simulink model "displayTest"  (R2022b)
settings: Solver=FixedStepDiscrete  StartTime=0.0  StopTime=10.0  FixedStep=0.01  RelTol=1e-3  EnableMultiTasking=on
PreLoadFcn:
  | try, model_open; catch, disp('Error occurred while executing model pre-load callback: model_open.m'); disp('Please assure that the MATLAB working directory is set to the model directory before opening.'); end
InitFcn:
  | try, model_open; catch, end
model workspace (MAT data in the model file):
  IOScreen_Label_XCoord = 1
  IOScreen_Row1_YCoord = 1
  IOScreen_Row2_YCoord = 12
  IOScreen_Value_XCoord = 110
  MainScreen_Row1_YCoord = 7
  MainScreen_Row2_YCoord = 23
  MainScreen_Symbols_XCoord = 1
  MainScreen_Units_XCoord = 69
  MainScreen_Value_XCoord = 64
undefined symbols (not defined in the file or in its folder): curr_screen, DISP, gesture, raptor_get_buildNum, raptor_get_safe_string, raptor_hwexp, raptor_xcp_function, Screens, VC500
libraries: Raptor_display_lib x93, Raptor_lib x40, Raptor_Datalogging_lib x10, simulink_extras x3, simulink x2
(part 2 of 3)

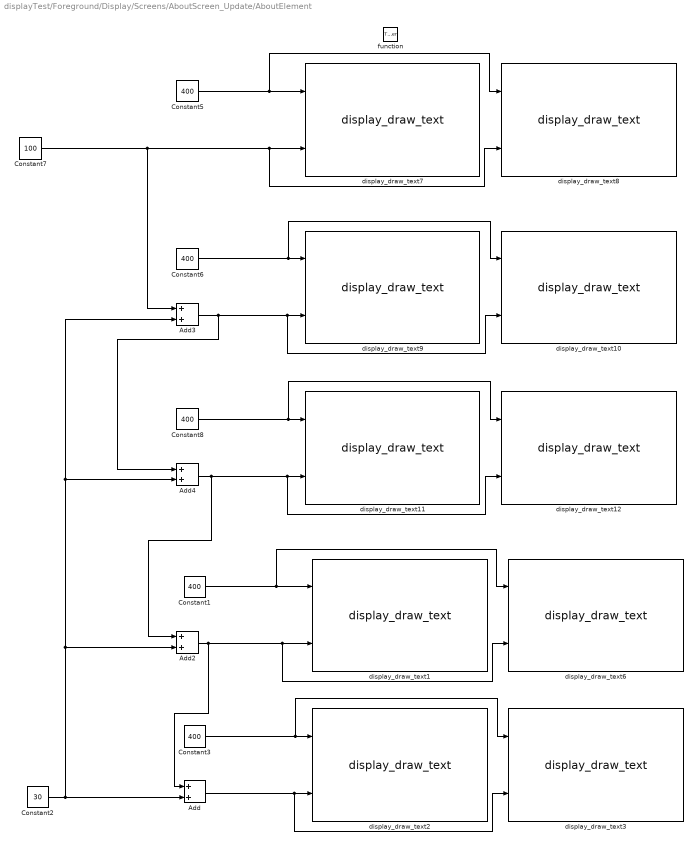
== system displayTest/Foreground/Display/Screens/AboutScreen_Update/AboutElement ==
  function : TriggerPort  TriggerType=function-call  VariantControl=Variant
  Add{,2..4} (4 alike) : Sum
  Constant{1,3,5..6,8} (5 alike) : Constant  Value=400  OutDataTypeStr=int32
  Constant2 : Constant  Value=30  OutDataTypeStr=int32
  Constant7 : Constant  Value=100  OutDataTypeStr=int32
  display_draw_text1 : Raptor_display_lib/Drawing Functions/display_draw_text  textPort=off  textVal='Raptor Version : '  colorPort=off  col=FFFF  opacity=100  font=Future  fontFile=''  heightPort=off  height=20  hAlign=Right  vAlign=Top  spacing=0  layer=Background  pnPort=off
      settings: SourceProductName=Raptor Display Library
  display_draw_text10 : Raptor_display_lib/Drawing Functions/display_draw_text  textPort=off  textVal=get_param(bdroot, 'ModelVersion')  colorPort=off  col=FFFF  opacity=100  font=Future  fontFile=''  heightPort=off  height=20  hAlign=Left  vAlign=Top  spacing=0  layer=Background  pnPort=off
      settings: SourceProductName=Raptor Display Library
  display_draw_text11 : Raptor_display_lib/Drawing Functions/display_draw_text  textPort=off  textVal='Build Number : '  colorPort=off  col=FFFF  opacity=100  font=Future  fontFile=''  heightPort=off  height=20  hAlign=Right  vAlign=Top  spacing=0  layer=Background  pnPort=off
      settings: SourceProductName=Raptor Display Library
  display_draw_text12 : Raptor_display_lib/Drawing Functions/display_draw_text  textPort=off  textVal=num2str(raptor_get_buildNum(bdroot(gcb)))  colorPort=off  col=FFFF  opacity=100  font=Future  fontFile=''  heightPort=off  height=20  hAlign=Left  vAlign=Top  spacing=0  layer=Background  pnPort=off
      settings: SourceProductName=Raptor Display Library
  display_draw_text2 : Raptor_display_lib/Drawing Functions/display_draw_text  textPort=off  textVal='MATLAB Version : '  colorPort=off  col=FFFF  opacity=100  font=Future  fontFile=''  heightPort=off  height=20  hAlign=Right  vAlign=Top  spacing=0  layer=Background  pnPort=off
      settings: SourceProductName=Raptor Display Library
  display_draw_text3 : Raptor_display_lib/Drawing Functions/display_draw_text  textPort=off  textVal=version  colorPort=off  col=FFFF  opacity=100  font=Future  fontFile=''  heightPort=off  height=20  hAlign=Left  vAlign=Top  spacing=0  layer=Background  pnPort=off
      settings: SourceProductName=Raptor Display Library
  display_draw_text6 : Raptor_display_lib/Drawing Functions/display_draw_text  textPort=off  textVal=raptor_hwexp('COMMAND:RAPTOR_VERSION')  colorPort=off  col=FFFF  opacity=100  font=Future  fontFile=''  heightPort=off  height=20  hAlign=Left  vAlign=Top  spacing=0  layer=Background  pnPort=off
      settings: SourceProductName=Raptor Display Library
  display_draw_text7 : Raptor_display_lib/Drawing Functions/display_draw_text  textPort=off  textVal='Application Name : '  colorPort=off  col=FFFF  opacity=100  font=Future  fontFile=''  heightPort=off  height=20  hAlign=Right  vAlign=Top  spacing=0  layer=Background  pnPort=off
      settings: SourceProductName=Raptor Display Library
  display_draw_text8 : Raptor_display_lib/Drawing Functions/display_draw_text  textPort=off  textVal=bdroot  colorPort=off  col=FFFF  opacity=100  font=Future  fontFile=''  heightPort=off  height=20  hAlign=Left  vAlign=Top  spacing=0  layer=Background  pnPort=off
      settings: SourceProductName=Raptor Display Library
  display_draw_text9 : Raptor_display_lib/Drawing Functions/display_draw_text  textPort=off  textVal='Model Version : '  colorPort=off  col=FFFF  opacity=100  font=Future  fontFile=''  heightPort=off  height=20  hAlign=Right  vAlign=Top  spacing=0  layer=Background  pnPort=off
      settings: SourceProductName=Raptor Display Library
  wires:
  Constant1/1 -> display_draw_text6/1, display_draw_text1/1
  Add/1 -> display_draw_text2/2, display_draw_text3/2
  Constant3/1 -> display_draw_text2/1, display_draw_text3/1
  Constant5/1 -> display_draw_text7/1, display_draw_text8/1
  Add2/1 -> Add/1, display_draw_text6/2, display_draw_text1/2
  Constant2/1 -> Add3/2, Add4/2, Add2/2, Add/2
  Add4/1 -> Add2/1, display_draw_text11/2, display_draw_text12/2
  Constant8/1 -> display_draw_text11/1, display_draw_text12/1
  Add3/1 -> Add4/1, display_draw_text9/2, display_draw_text10/2
  Constant6/1 -> display_draw_text9/1, display_draw_text10/1
  Constant7/1 -> display_draw_text7/2, display_draw_text8/2, Add3/1

== system displayTest/Foreground/Display/Screens/DataLogScreen_Create/DataLogScreenSwipe ==
  note: This function is called when a swipe action occurs.  The gesture input will
      |  provide the gesture detected:
      |   0 = UP
      |   1 = DOWN
      |   2 = LEFT
      |   3 = RIGHT
  DataLogScreenSwipe : TriggerPort  TriggerType=function-call  IsSimulinkFunction=on  FunctionName=DataLogScreenSwipe  FunctionVisibility=scoped  VariantControl=Variant  PortDimensions=1
  Constant : Constant  Value=3  OutDataTypeStr=uint8
  Function Caller : FunctionCaller  FunctionPrototype=Screens.Navigation(gesture,curr_screen)  InputArgumentSpecifications=<Enter example>  OutputArgumentSpecifications=<Enter example>
  gesture : ArgIn  OutDataTypeStr=uint8  ArgumentName=gesture
  wires:
  gesture/1 -> Function Caller/1
  Constant/1 -> Function Caller/2

== system displayTest/Foreground/Display/Screens/DataLogScreen_CurrentScreen/EjectButtonPressed ==
  Trigger : TriggerPort  TriggerType=falling  VariantControl=Variant  PortDimensions=1
  raptor_fileIO_USBEject : Raptor_Datalogging_lib/raptor_fileIO_USBEject  variable=0
      settings: SourceProductName=Raptor Data Logging

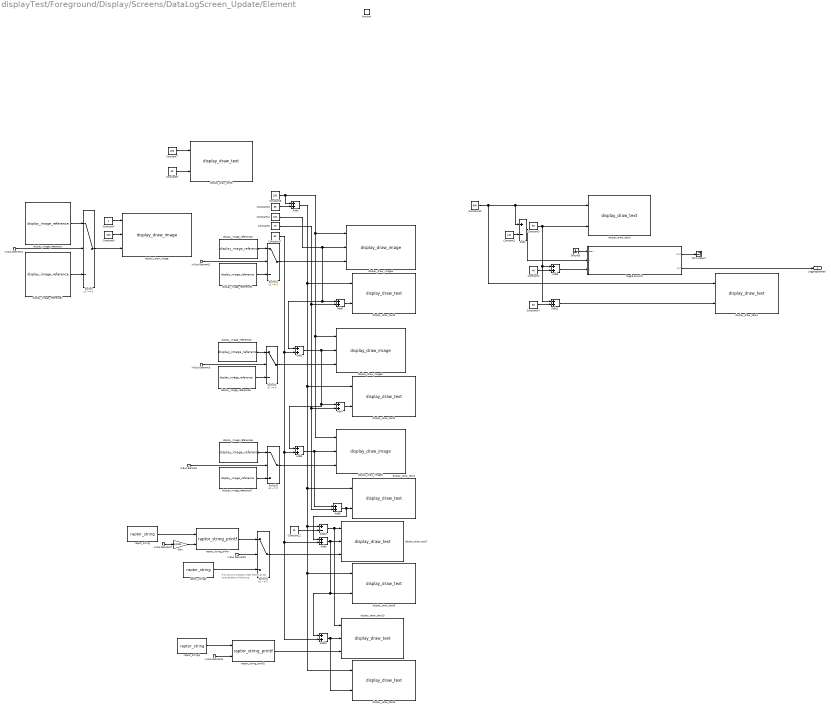
== system displayTest/Foreground/Display/Screens/DataLogScreen_Update/Element ==
  note: If no drive is present, then there can
      | be no evaluation of the size
  In Bus Element2 : Inport  PortName=DataLogState  Element=LoggingPossible
  In Bus Element3 : Inport  PortName=DataLogState  Element=LoggingActive
  In Bus Element : Inport  PortName=DataLogState  Element=EjectReady
  In Bus Element1 : Inport  PortName=DataLogState  Element=USBInserted
  In Bus Element5 : Inport  PortName=DataLogState  Element=USBInserted
  In Bus Element4 : Inport  PortName=DataLogState  Element=LogCounter
  In Bus Element7 : Inport  Port=2  PortName=Sensors  Element=USBFreeSpace
  function : TriggerPort  TriggerType=function-call  VariantControl=Variant
  Add{1,3..9,11,13} (10 alike) : Sum
  Add10 : Sum  Inputs=+-
  Add2 : Sum  Inputs=+-
  Constant1 : Constant  Value=140  OutDataTypeStr=int32
  Constant10 : Constant  Value=600  OutDataTypeStr=int32
  Constant11 : Constant  Value=100  OutDataTypeStr=int32
  Constant12 : Constant  Value=15  OutDataTypeStr=int32
  Constant13 : Constant  Value=65  OutDataTypeStr=int32
  Constant14 : Constant  Value=50  OutDataTypeStr=int32
  Constant17 : Constant  Value=60  OutDataTypeStr=int32
  Constant2 : Constant  Value=40  OutDataTypeStr=int32
  Constant3 : Constant  Value=50  OutDataTypeStr=int32
  Constant4 : Constant  OutDataTypeStr=int32
  Constant5 : Constant  Value=19  OutDataTypeStr=int32
  Constant6 : Constant  Value=100  OutDataTypeStr=int32
  Constant7 : Constant  Value=200  OutDataTypeStr=int32
  Constant8 : Constant  Value=150  OutDataTypeStr=int32
  Constant9 : Constant  Value=50  OutDataTypeStr=int32
  Gain : Gain  Gain=1/1024  OutDataTypeStr=uint32
  Ground3 : Ground
  Switch{,1..4} (5 alike) : Switch  Criteria=u2 ~= 0  SaturateOnIntegerOverflow=off  InputSameDT=off
  Terminator2 : Terminator
  Toggle Switch1 : Subsystem  mask(Display Toggle){InitialCondition=0}
      mask prompts: InitialCondition "Initial Condition"
      mask help: Draws a toggle switch onto the screen that will hold either an off or an on state
      mask Help: eval('raptor_display_help(''Toggle Switch'');')
      mask Display:
      | header = 'Toggle Switch';
      | drawNEBackGndDisplay;
      | port_label('input', 1, 'prev');
      | port_label('input', 2, 'x[int32]');
      | port_label('input', 3, 'y[int32]');
      | port_label('output', 1, 'next');
      | port_label('output', 2, 'out[boolean]');
      | 
      | image(imread('toggle_frame.png'), [0.3 0.2 0.3 0.34]);
  display_draw_image{,1..3} (4 alike) : Raptor_display_lib/Drawing Functions/display_draw_image  imagePort=on  imageFile=USB_Icon_Sprite_Green_25perc.png  opacityPort=off  opacity=100  drawMode=Draw Entire Image  alpha=Draw as Transparent  layer=Background  drawModeXY=Top Left  pnPort=off
      settings: SourceProductName=Raptor Display Library
  display_draw_text1 : Raptor_display_lib/Drawing Functions/display_draw_text  textPort=off  textVal='Ready to Eject'  colorPort=off  col=FFFF  opacity=100  font=Future  fontFile=''  heightPort=off  height=20  hAlign=Left  vAlign=Top  spacing=0  layer=Background  pnPort=off
      settings: SourceProductName=Raptor Display Library
  display_draw_text10 : Raptor_display_lib/Drawing Functions/display_draw_text  textPort=on  textVal='Eject Ready'  colorPort=off  col=FFFF  opacity=100  font=Future  fontFile=''  heightPort=off  height=20  hAlign=Right  vAlign=Top  spacing=0  layer=Background  pnPort=off
      settings: SourceProductName=Raptor Display Library
  display_draw_text2 : Raptor_display_lib/Drawing Functions/display_draw_text  textPort=off  textVal='Control'  colorPort=off  col=FFFF  opacity=100  font=Future  fontFile=''  heightPort=off  height=30  hAlign=Center  vAlign=Top  spacing=0  layer=Background  pnPort=off
      settings: SourceProductName=Raptor Display Library
  display_draw_text3 : Raptor_display_lib/Drawing Functions/display_draw_text  textPort=off  textVal='Logging Active'  colorPort=off  col=FFFF  opacity=100  font=Future  fontFile=''  heightPort=off  height=20  hAlign=Left  vAlign=Top  spacing=0  layer=Background  pnPort=off
      settings: SourceProductName=Raptor Display Library
  display_draw_text4 : Raptor_display_lib/Drawing Functions/display_draw_text  textPort=off  textVal='Logging'  colorPort=off  col=FFFF  opacity=100  font=Future  fontFile=''  heightPort=off  height=20  hAlign=Left  vAlign=Top  spacing=0  layer=Background  pnPort=off
      settings: SourceProductName=Raptor Display Library
  display_draw_text5 : Raptor_display_lib/Drawing Functions/display_draw_text  textPort=off  textVal='Ready to Log'  colorPort=off  col=FFFF  opacity=100  font=Future  fontFile=''  heightPort=off  height=20  hAlign=Left  vAlign=Top  spacing=0  layer=Background  pnPort=off
      settings: SourceProductName=Raptor Display Library
  display_draw_text6 : Raptor_display_lib/Drawing Functions/display_draw_text  textPort=off  textVal='USB Free Space'  colorPort=off  col=FFFF  opacity=100  font=Future  fontFile=''  heightPort=off  height=20  hAlign=Left  vAlign=Top  spacing=0  layer=Background  pnPort=off
      settings: SourceProductName=Raptor Display Library
  display_draw_text7 : Raptor_display_lib/Drawing Functions/display_draw_text  textPort=on  textVal='Eject Ready'  colorPort=off  col=FFFF  opacity=100  font=Future  fontFile=''  heightPort=off  height=20  hAlign=Right  vAlign=Top  spacing=0  layer=Background  pnPort=off
      settings: SourceProductName=Raptor Display Library
  display_draw_text8 : Raptor_display_lib/Drawing Functions/display_draw_text  textPort=off  textVal='Status'  colorPort=off  col=FFFF  opacity=100  font=Future  fontFile=''  heightPort=off  height=30  hAlign=Center  vAlign=Top  spacing=0  layer=Background  pnPort=off
      settings: SourceProductName=Raptor Display Library
  display_draw_text9 : Raptor_display_lib/Drawing Functions/display_draw_text  textPort=off  textVal='# Lines Logged'  colorPort=off  col=FFFF  opacity=100  font=Future  fontFile=''  heightPort=off  height=20  hAlign=Left  vAlign=Top  spacing=0  layer=Background  pnPort=off
      settings: SourceProductName=Raptor Display Library
  display_image_reference : Raptor_display_lib/Drawing Functions/display_image_reference  imageFile=USB_Icon_Sprite_Green_25perc.png
      settings: SourceProductName=Raptor Display Library
  display_image_reference1 : Raptor_display_lib/Drawing Functions/display_image_reference  imageFile=USB_Icon_Sprite_Red_25perc.png
      settings: SourceProductName=Raptor Display Library
  display_image_reference2 : Raptor_display_lib/Drawing Functions/display_image_reference  imageFile=Oval Driver@2x.png
      settings: SourceProductName=Raptor Display Library
  display_image_reference3 : Raptor_display_lib/Drawing Functions/display_image_reference  imageFile=Oval Active@2x.png
      settings: SourceProductName=Raptor Display Library
  display_image_reference4 : Raptor_display_lib/Drawing Functions/display_image_reference  imageFile=Oval Driver@2x.png
      settings: SourceProductName=Raptor Display Library
  display_image_reference5 : Raptor_display_lib/Drawing Functions/display_image_reference  imageFile=Oval Active@2x.png
      settings: SourceProductName=Raptor Display Library
  display_image_reference6 : Raptor_display_lib/Drawing Functions/display_image_reference  imageFile=Oval Driver@2x.png
      settings: SourceProductName=Raptor Display Library
  display_image_reference7 : Raptor_display_lib/Drawing Functions/display_image_reference  imageFile=Oval Active@2x.png
      settings: SourceProductName=Raptor Display Library
  raptor_string : Raptor_lib/Strings/raptor_string  stringName=''  string=''  dynamicSize=Fixed Size  strSize=20  storage=Volatile (RAM)  calVisible=off  calAccess=4  strFunction=raptor_xcp_function(gcb)
      settings: SourceProductName=Raptor
  raptor_string1 : Raptor_lib/Strings/raptor_string  stringName=''  string=''  dynamicSize=Fixed Size  strSize=20  storage=Volatile (RAM)  calVisible=off  calAccess=4  strFunction=raptor_xcp_function(gcb)
      settings: SourceProductName=Raptor
  raptor_string2 : Raptor_lib/Strings/raptor_string  stringName=''  string='N/A'  dynamicSize=Size from initial value  strSize=20  storage=Volatile (RAM)  calVisible=off  calAccess=4  strFunction=raptor_xcp_function(gcb)
      settings: SourceProductName=Raptor
  raptor_string_printf : Raptor_lib/Strings/raptor_string_printf  formatString='%u KB'
      settings: SourceProductName=Raptor
  raptor_string_printf1 : Raptor_lib/Strings/raptor_string_printf  formatString='%u'
      settings: SourceProductName=Raptor
  LoggingEnabled : Outport  VectorParamsAs1DForOutWhenUnconnected=off
  wires:
  Constant2/1 -> Add3/2
  Add2/1 -> Toggle Switch1/2(x)
  Toggle Switch1/1(next) -> Terminator2/1
  Toggle Switch1/2(out) -> LoggingEnabled/1
  Ground3/1 -> Toggle Switch1/1(prev)
  Constant10/1 -> display_draw_text4/1, Add2/1, display_draw_text2/1
  Constant1/1 -> Add2/2
  Add3/1 -> Toggle Switch1/3(y)
  Constant6/1 -> display_draw_image/2
  Constant4/1 -> display_draw_image/1
  display_image_reference/1 -> Switch/1
  display_image_reference1/1 -> Switch/3
  In Bus Element1/1 -> Switch/2
  Switch/1 -> display_draw_image/3
  Switch1/1 -> display_draw_image1/3
  Constant8/1 -> Add4/1, display_draw_image3/1, display_draw_image2/1, display_draw_image1/1
  Constant11/1 -> Add1/1, Add6/1, display_draw_image1/2
  Add1/1 -> Add7/1, Add5/1, display_draw_image2/2
  Switch2/1 -> display_draw_image2/3
  Switch3/1 -> display_draw_image3/3
  display_image_reference7/1 -> Switch3/3
  display_image_reference6/1 -> Switch3/1
  In Bus Element/1 -> Switch3/2
  Constant13/1 -> Add4/2
  Constant17/1 -> Add13/2, Add9/2, Add5/2, Add1/2
  Add5/1 -> Add8/1, display_draw_image3/2
  Constant5/1 -> Add8/2, Add7/2, Add6/2
  Add6/1 -> display_draw_text5/2
  Add7/1 -> display_draw_text3/2
  Add8/1 -> Add9/1, display_draw_text1/2
  raptor_string/1 -> raptor_string_printf/1
  In Bus Element7/1 -> Gain/1
  Constant7/1 -> display_draw_text8/1
  Constant9/1 -> display_draw_text8/2
  Constant12/1 -> Add10/2
  Constant3/1 -> Add11/1, Add3/1, display_draw_text2/2
  Add10/1 -> display_draw_text10/1, display_draw_text7/1
  Add13/1 -> display_draw_text10/2, display_draw_text9/2
  raptor_string_printf1/1 -> display_draw_text10/3
  In Bus Element4/1 -> raptor_string_printf1/2
  raptor_string1/1 -> raptor_string_printf1/1
  Add9/1 -> Add13/1, display_draw_text6/2, display_draw_text7/2
  Add4/1 -> display_draw_text5/1, Add10/1, display_draw_text9/1, display_draw_text6/1, display_draw_text1/1, display_draw_text3/1
  raptor_string_printf/1 -> Switch4/1
  Switch4/1 -> display_draw_text7/3
  raptor_string2/1 -> Switch4/3
  In Bus Element5/1 -> Switch4/2
  Gain/1 -> raptor_string_printf/2
  In Bus Element3/1 -> Switch2/2
  display_image_reference4/1 -> Switch2/1
  display_image_reference5/1 -> Switch2/3
  display_image_reference3/1 -> Switch1/3
  display_image_reference2/1 -> Switch1/1
  In Bus Element2/1 -> Switch1/2
  Add11/1 -> display_draw_text4/2
  Constant14/1 -> Add11/2

== system displayTest/Foreground/Display/Screens/IOScreen_Create/IOScreenSwipe ==
  note: This function is called when a swipe action occurs.  The gesture input will
      |  provide the gesture detected:
      |   0 = UP
      |   1 = DOWN
      |   2 = LEFT
      |   3 = RIGHT
  IOScreenSwipe : TriggerPort  TriggerType=function-call  IsSimulinkFunction=on  FunctionName=IOScreenSwipe  FunctionVisibility=scoped  VariantControl=Variant  PortDimensions=1
  Constant : Constant  Value=2  OutDataTypeStr=uint8
  Function Caller : FunctionCaller  FunctionPrototype=Screens.Navigation(gesture,curr_screen)  InputArgumentSpecifications=<Enter example>  OutputArgumentSpecifications=<Enter example>
  gesture : ArgIn  OutDataTypeStr=uint8  ArgumentName=gesture
  wires:
  Constant/1 -> Function Caller/2
  gesture/1 -> Function Caller/1

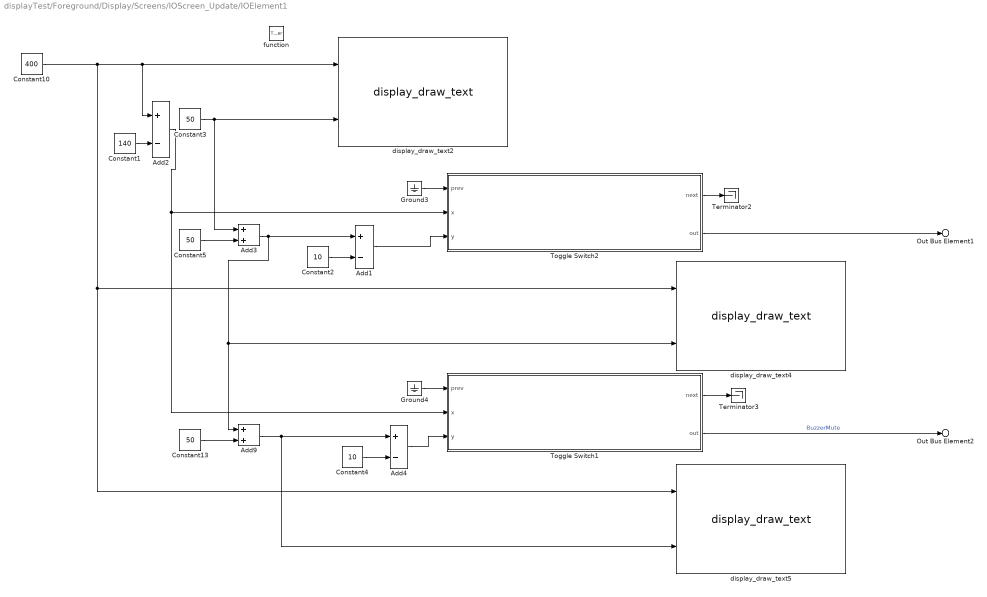
== system displayTest/Foreground/Display/Screens/IOScreen_Update/IOElement1 ==
  function : TriggerPort  TriggerType=function-call  VariantControl=Variant
  Add1 : Sum  Inputs=+-
  Add2 : Sum  Inputs=+-
  Add3 : Sum
  Add4 : Sum  Inputs=+-
  Add9 : Sum
  Constant1 : Constant  Value=140  OutDataTypeStr=int32
  Constant10 : Constant  Value=400  OutDataTypeStr=int32
  Constant13 : Constant  Value=50  OutDataTypeStr=int32
  Constant2 : Constant  Value=10  OutDataTypeStr=int32
  Constant3 : Constant  Value=50  OutDataTypeStr=int32
  Constant4 : Constant  Value=10  OutDataTypeStr=int32
  Constant5 : Constant  Value=50  OutDataTypeStr=int32
  Ground3 : Ground
  Ground4 : Ground
  Terminator2 : Terminator
  Terminator3 : Terminator
  Toggle Switch1 : Subsystem  mask(Display Toggle){InitialCondition=0}
      mask prompts: InitialCondition "Initial Condition"
      mask help: Draws a toggle switch onto the screen that will hold either an off or an on state
      mask Help: eval('raptor_display_help(''Toggle Switch'');')
      mask Display:
      | header = 'Toggle Switch';
      | drawNEBackGndDisplay;
      | port_label('input', 1, 'prev');
      | port_label('input', 2, 'x[int32]');
      | port_label('input', 3, 'y[int32]');
      | port_label('output', 1, 'next');
      | port_label('output', 2, 'out[boolean]');
      | 
      | image(imread('toggle_frame.png'), [0.3 0.2 0.3 0.34]);
  Toggle Switch2 : Subsystem  mask(Display Toggle){InitialCondition=0}
      mask prompts: InitialCondition "Initial Condition"
      mask help: Draws a toggle switch onto the screen that will hold either an off or an on state
      mask Help: eval('raptor_display_help(''Toggle Switch'');')
      mask Display:
      | header = 'Toggle Switch';
      | drawNEBackGndDisplay;
      | port_label('input', 1, 'prev');
      | port_label('input', 2, 'x[int32]');
      | port_label('input', 3, 'y[int32]');
      | port_label('output', 1, 'next');
      | port_label('output', 2, 'out[boolean]');
      | 
      | image(imread('toggle_frame.png'), [0.3 0.2 0.3 0.34]);
  display_draw_text2 : Raptor_display_lib/Drawing Functions/display_draw_text  textPort=off  textVal='Outputs'  colorPort=off  col=FFFF  opacity=100  font=Future  fontFile=''  heightPort=off  height=30  hAlign=Center  vAlign=Top  spacing=0  layer=Background  pnPort=off
      settings: SourceProductName=Raptor Display Library
  display_draw_text4 : Raptor_display_lib/Drawing Functions/display_draw_text  textPort=off  textVal='Buzzer'  colorPort=off  col=FFFF  opacity=100  font=Future  fontFile=''  heightPort=off  height=20  hAlign=Left  vAlign=Top  spacing=0  layer=Background  pnPort=off
      settings: SourceProductName=Raptor Display Library
  display_draw_text5 : Raptor_display_lib/Drawing Functions/display_draw_text  textPort=off  textVal='Buzzer Mute'  colorPort=off  col=FFFF  opacity=100  font=Future  fontFile=''  heightPort=off  height=20  hAlign=Left  vAlign=Top  spacing=0  layer=Background  pnPort=off
      settings: SourceProductName=Raptor Display Library
  Out Bus Element1 : Outport  VectorParamsAs1DForOutWhenUnconnected=off  PortName=Actuators  Element=Buzzer
  Out Bus Element2 : Outport  VectorParamsAs1DForOutWhenUnconnected=off  PortName=Actuators  Element=BuzzerMute
  wires:
  Constant13/1 -> Add9/2
  Ground4/1 -> Toggle Switch1/1(prev)
  Add9/1 -> Add4/1, display_draw_text5/2
  Toggle Switch1/1(next) -> Terminator3/1
  Toggle Switch1/2(out) -> Out Bus Element2/1  "BuzzerMute"
  Toggle Switch2/2(out) -> Out Bus Element1/1
  Toggle Switch2/1(next) -> Terminator2/1
  Ground3/1 -> Toggle Switch2/1(prev)
  Constant10/1 -> Add2/1, display_draw_text2/1, display_draw_text4/1, display_draw_text5/1
  Constant3/1 -> Add3/1, display_draw_text2/2
  Add2/1 -> Toggle Switch2/2(x), Toggle Switch1/2(x)
  Constant1/1 -> Add2/2
  Add3/1 -> Add1/1, display_draw_text4/2, Add9/1
  Constant5/1 -> Add3/2
  Constant2/1 -> Add1/2
  Add1/1 -> Toggle Switch2/3(y)
  Constant4/1 -> Add4/2
  Add4/1 -> Toggle Switch1/3(y)

== system displayTest/Foreground/Display/Screens/MainScreen_Create/MainScreenSwipe ==
  note: This function is called when a swipe action occurs.  The gesture input will
      |  provide the gesture detected:
      |   0 = UP
      |   1 = DOWN
      |   2 = LEFT
      |   3 = RIGHT
  MainScreenSwipe : TriggerPort  TriggerType=function-call  IsSimulinkFunction=on  FunctionName=MainScreenSwipe  FunctionVisibility=scoped  VariantControl=Variant  PortDimensions=1
  Constant : Constant  OutDataTypeStr=uint8
  Function Caller : FunctionCaller  FunctionPrototype=Screens.Navigation(gesture,curr_screen)  InputArgumentSpecifications=<Enter example>  OutputArgumentSpecifications=<Enter example>
  gesture : ArgIn  OutDataTypeStr=uint8  ArgumentName=gesture
  wires:
  gesture/1 -> Function Caller/1
  Constant/1 -> Function Caller/2

== system displayTest/Foreground/Display/Screens/MainScreen_Update/Illumination Invalid ==
  Xbase : Inport
  Ybase : Inport  Port=2
  Prev : Inport  Port=3
  Enable : EnablePort
  Add : Sum
  Add1 : Sum  Inputs=+-
  Constant1 : Constant  Value=51  OutDataTypeStr=int32
  Constant74 : Constant  Value=20  OutDataTypeStr=int32
  Terminator : Terminator
  display_draw_image : Raptor_display_lib/Drawing Functions/display_draw_image  imagePort=off  imageFile=FaultRED.bmp  opacityPort=off  opacity=100  drawMode=Draw Entire Image  alpha=Draw as Transparent  layer=Background  drawModeXY=Top Left  pnPort=on
      settings: SourceProductName=Raptor Display Library
  wires:
  display_draw_image/1 -> Terminator/1
  Prev/1 -> display_draw_image/1
  Add/1 -> display_draw_image/3
  Constant74/1 -> Add/2
  Ybase/1 -> Add/1
  Constant1/1 -> Add1/2
  Xbase/1 -> Add1/1
  Add1/1 -> display_draw_image/2

== system displayTest/Foreground/Display/Screens/MainScreen_Update/RPM Invalid ==
  Xbase : Inport
  Ybase : Inport  Port=2
  Prev : Inport  Port=3
  Enable : EnablePort
  Add : Sum
  Constant74 : Constant  Value=20  OutDataTypeStr=int32
  Terminator : Terminator
  display_draw_image : Raptor_display_lib/Drawing Functions/display_draw_image  imagePort=off  imageFile=FaultRED.bmp  opacityPort=off  opacity=100  drawMode=Draw Entire Image  alpha=Draw as Transparent  layer=Background  drawModeXY=Top Left  pnPort=on
      settings: SourceProductName=Raptor Display Library
  wires:
  Xbase/1 -> display_draw_image/2
  Ybase/1 -> Add/1
  Constant74/1 -> Add/2
  Add/1 -> display_draw_image/3
  Prev/1 -> display_draw_image/1
  display_draw_image/1 -> Terminator/1

== system displayTest/Foreground/Display/Screens/Navigation/Go Left ==
  Current Screen : Inport
  Action Port : ActionPort  ActionPortLabel=elseif(u1 == 2)
  About : Subsystem  TreatAsAtomicUnit=on
  DataLog : Subsystem  TreatAsAtomicUnit=on
  Default : Subsystem  TreatAsAtomicUnit=on
  IO : Subsystem  TreatAsAtomicUnit=on
  Main : Subsystem  TreatAsAtomicUnit=on
  Switch Case1 : SwitchCase  CaseConditions={1,2,3,4}
  wires:
  Switch Case1/2 -> IO/Action
  Switch Case1/5 -> Default/Action
  Switch Case1/4 -> About/Action
  Switch Case1/1 -> Main/Action
  Switch Case1/3 -> DataLog/Action
  Current Screen/1 -> Switch Case1/1

== system displayTest/Foreground/Display/Screens/Navigation/Go Right ==
  Current Screen : Inport
  Action Port : ActionPort  ActionPortLabel=if(u1 == 3)
  About : Subsystem  TreatAsAtomicUnit=on
  DataLog : Subsystem  TreatAsAtomicUnit=on
  Default : Subsystem  TreatAsAtomicUnit=on
  IO : Subsystem  TreatAsAtomicUnit=on
  Main : Subsystem  TreatAsAtomicUnit=on
  Switch Case : SwitchCase  CaseConditions={1,2,3,4}
  wires:
  Current Screen/1 -> Switch Case/1
  Switch Case/1 -> Main/Action
  Switch Case/3 -> DataLog/Action
  Switch Case/4 -> About/Action
  Switch Case/2 -> IO/Action
  Switch Case/5 -> Default/Action

== system displayTest/Foreground/Display/Screens/Navigation/Go Up or Down ==
  note: Do Nothing when a "UP" or "DOWN" is performed
  Current Screen : Inport
  Action Port : ActionPort  ActionPortLabel=else
  Terminator : Terminator
  wires:
  Current Screen/1 -> Terminator/1

== system displayTest/Foreground/Plant/Inputs/J1939 Rx/Process Illumination Message ==
  note: default to 100% illumination
  note: timeout occurred
  note: new message
  AgeCount : Inport
  Data : Inport  Port=2
  Constant : Constant  Value=750
  Constant1 : Constant  Value=0
  Constant2 : Constant  Value=100
  Constant3 : Constant  Value=100
  Logical Operator : Logic  Operator=NOT  AllPortsSameDT=off  OutDataTypeStr=boolean
  Logical Operator1 : Logic  Operator=OR  AllPortsSameDT=off  OutDataTypeStr=boolean
  Relational Operator : RelationalOperator  Operator=>  OutDataTypeStr=boolean  RndMeth=Simplest  InputSameDT=off
  Relational Operator1 : RelationalOperator  Operator===  OutDataTypeStr=boolean  RndMeth=Simplest  InputSameDT=off
  Relational Operator2 : RelationalOperator  Operator=>  OutDataTypeStr=boolean  RndMeth=Simplest  InputSameDT=off
  Switch : Switch  Criteria=u2 ~= 0  SaturateOnIntegerOverflow=off  InputSameDT=off
  Switch1 : Switch  Criteria=u2 ~= 0  SaturateOnIntegerOverflow=off  InputSameDT=off
  Unit Delay : UnitDelay  SampleTime=-1  HasFrameUpgradeWarning=on
  Illumination : Outport  VectorParamsAs1DForOutWhenUnconnected=off
  IlluminationValid : Outport  Port=2  VectorParamsAs1DForOutWhenUnconnected=off
  wires:
  Constant/1 -> Relational Operator/2
  Logical Operator/1 -> IlluminationValid/1
  Switch/1 -> Illumination/1, Unit Delay/1
  AgeCount/1 -> Relational Operator1/1, Relational Operator/1
  Constant1/1 -> Relational Operator1/2
  Relational Operator1/1 -> Switch1/2
  Data/1 -> Switch1/1, Relational Operator2/1
  Switch1/1 -> Switch/3
  Unit Delay/1 -> Switch1/3
  Constant2/1 -> Switch/1
  Relational Operator/1 -> Logical Operator1/1
  Logical Operator1/1 -> Switch/2, Logical Operator/1
  Relational Operator2/1 -> Logical Operator1/2
  Constant3/1 -> Relational Operator2/2

== system displayTest/Foreground/Plant/Inputs/J1939 Rx/Process RPM Message ==
  note: timeout occurred
  note: new message
  AgeCount : Inport
  Data : Inport  Port=2
  Constant : Constant  Value=100
  Constant1 : Constant  Value=0
  Constant2 : Constant  Value=0
  Constant3 : Constant  Value=8031.88
  Logical Operator : Logic  Operator=NOT  AllPortsSameDT=off  OutDataTypeStr=boolean
  Logical Operator1 : Logic  Operator=OR  AllPortsSameDT=off  OutDataTypeStr=boolean
  Relational Operator : RelationalOperator  Operator=>  OutDataTypeStr=boolean  RndMeth=Simplest  InputSameDT=off
  Relational Operator1 : RelationalOperator  Operator===  OutDataTypeStr=boolean  RndMeth=Simplest  InputSameDT=off
  Relational Operator2 : RelationalOperator  Operator=>  OutDataTypeStr=boolean  RndMeth=Simplest  InputSameDT=off
  Switch : Switch  Criteria=u2 ~= 0  SaturateOnIntegerOverflow=off  InputSameDT=off
  Switch1 : Switch  Criteria=u2 ~= 0  SaturateOnIntegerOverflow=off  InputSameDT=off
  Unit Delay : UnitDelay  SampleTime=-1  HasFrameUpgradeWarning=on
  EngineRPM : Outport  VectorParamsAs1DForOutWhenUnconnected=off
  EngineRPMValid : Outport  Port=2  VectorParamsAs1DForOutWhenUnconnected=off
  wires:
  Constant/1 -> Relational Operator/2
  Logical Operator/1 -> EngineRPMValid/1
  Switch/1 -> EngineRPM/1, Unit Delay/1
  AgeCount/1 -> Relational Operator1/1, Relational Operator/1
  Constant1/1 -> Relational Operator1/2
  Relational Operator1/1 -> Switch1/2
  Data/1 -> Switch1/1, Relational Operator2/1
  Switch1/1 -> Switch/3
  Unit Delay/1 -> Switch1/3
  Constant2/1 -> Switch/1
  Relational Operator/1 -> Logical Operator1/1
  Logical Operator1/1 -> Switch/2, Logical Operator/1
  Relational Operator2/1 -> Logical Operator1/2
  Constant3/1 -> Relational Operator2/2

== system displayTest/Foreground/Display/Data Logging/Write to Log/File Write Action/Sync File ==
  In1 : Inport
  Enable : EnablePort
  Terminator : Terminator
  Terminator1 : Terminator
  raptor_data_write : Raptor_lib/Data Storage/raptor_data_write  dataName='LastSync'  dataShape=Scalar  idxSource=Input Port  idxRow=1  idxCol=1
      settings: SourceProductName=Raptor
  raptor_fileIO_sync1 : Raptor_Datalogging_lib/raptor_fileIO_sync  resourceValues=USB|(None)  resource=USB
      settings: SourceProductName=Raptor Data Logging
  raptor_time : Raptor_lib/Triggers/raptor_time  unit=milliseconds
      settings: SourceProductName=Raptor
  wires:
  raptor_time/1 -> raptor_data_write/1
  raptor_fileIO_sync1/1 -> Terminator/1
  In1/1 -> raptor_fileIO_sync1/1
  raptor_fileIO_sync1/2 -> Terminator1/1

== system displayTest/Foreground/Display/Data Logging/Write to Log/File Write Action/Sync every 10 Seconds ==
  Add1 : Sum  Inputs=+-
  Constant : Constant  Value=10000
  Logical Operator : Logic  Operator=OR  AllPortsSameDT=off  OutDataTypeStr=boolean
  Relational Operator : RelationalOperator  Operator=>  OutDataTypeStr=boolean  InputSameDT=off
  Relational Operator1 : RelationalOperator  Operator=<  OutDataTypeStr=boolean  InputSameDT=off
  Unit Delay : UnitDelay  SampleTime=-1  HasFrameUpgradeWarning=on
  raptor_data_def : Raptor_lib/Data Storage/raptor_data_def  dataName='LastSync'  initValue=0  dataType=uint32  storage=Volatile (RAM)  calVisible=on  calType=Measurement  calDispType=Number  calEnum={'False', 'True'}  calGain=1.0  calOffset=0  calMin=-Inf  calMax=Inf  calFormat='4.2'  calUnit=''  calHelp=['Block:' gcb]  calAccess=4  calFunction=raptor_xcp_function(gcb)  calDispHeaders=off  calColHeaders={'Col1' 'Col2' 'Col3'}  calRowHeaders={'Row1' 'Row2' 'Row3'}
      settings: SourceProductName=Raptor
  raptor_data_read1 : Raptor_lib/Data Storage/raptor_data_read  dataName='LastSync'  dataShape=Scalar  idxSource=Input  idxRow=1  idxCol=1
      settings: SourceProductName=Raptor
  raptor_time : Raptor_lib/Triggers/raptor_time  unit=milliseconds
      settings: SourceProductName=Raptor
  TimeToSync : Outport  VectorParamsAs1DForOutWhenUnconnected=off
  wires:
  Logical Operator/1 -> TimeToSync/1
  Relational Operator1/1 -> Logical Operator/2  "Rollover"
  Relational Operator/1 -> Logical Operator/1
  Constant/1 -> Relational Operator/2
  Add1/1 -> Relational Operator/1
  raptor_data_read1/1 -> Add1/2
  Unit Delay/1 -> Relational Operator1/2
  raptor_time/1 -> Relational Operator1/1, Add1/1, Unit Delay/1

== system displayTest/Foreground/Display/Data Logging/Write to Log/Open Existing File/File Seek ==
  Open File Handle : Inport
  Open Success : Inport  Port=2
  File Open Failure : Subsystem
  File Open Success : Subsystem
  Logical Operator : Logic  Operator=NOT  AllPortsSameDT=off  OutDataTypeStr=boolean
  Seek File Handle Success : Outport  VectorParamsAs1DForOutWhenUnconnected=off
  Seek Success : Outport  Port=2  VectorParamsAs1DForOutWhenUnconnected=off
  Seek File Handle Failure : Outport  Port=3  VectorParamsAs1DForOutWhenUnconnected=off
  Seek Failure : Outport  Port=4  VectorParamsAs1DForOutWhenUnconnected=off
  wires:
  Open File Handle/1 -> File Open Success/1(file_in), File Open Failure/1(file_in)
  Logical Operator/1 -> File Open Failure/Enable
  Open Success/1 -> Logical Operator/1, File Open Success/Enable
  File Open Success/1(file_out) -> Seek File Handle Success/1
  File Open Success/2(Out2) -> Seek Success/1
  File Open Failure/1(file_out) -> Seek File Handle Failure/1
  File Open Failure/2(Success) -> Seek Failure/1

== system displayTest/Foreground/Display/Data Logging/Write to Log/Open Existing File/Merge ==
  File Handle Success : Inport
  File Open Success : Inport  Port=2
  File Handle Failure : Inport  Port=3
  File Open Failure : Inport  Port=4
  Merge : Merge
  Merge1 : Merge
  Handle : Outport  VectorParamsAs1DForOutWhenUnconnected=off
  Success : Outport  Port=2  VectorParamsAs1DForOutWhenUnconnected=off
  wires:
  Merge1/1 -> Handle/1
  Merge/1 -> Success/1
  File Open Failure/1 -> Merge/2
  File Handle Failure/1 -> Merge1/2
  File Handle Success/1 -> Merge1/1
  File Open Success/1 -> Merge/1

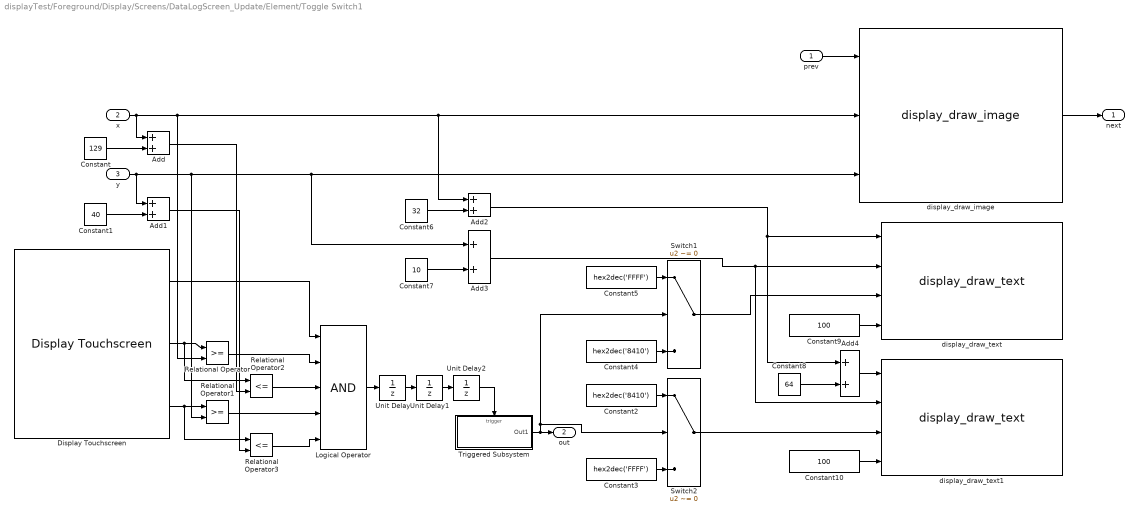
== system displayTest/Foreground/Display/Screens/DataLogScreen_Update/Element/Toggle Switch1 ==
  prev : Inport
  x : Inport  Port=2
  y : Inport  Port=3
  Add{,1..4} (5 alike) : Sum
  Constant : Constant  Value=129
  Constant1 : Constant  Value=40
  Constant10 : Constant  Value=100  OutDataTypeStr=uint32
  Constant2 : Constant  Value=hex2dec('8410')  OutDataTypeStr=uint16
  Constant3 : Constant  Value=hex2dec('FFFF')  OutDataTypeStr=uint16
  Constant4 : Constant  Value=hex2dec('8410')  OutDataTypeStr=uint16
  Constant5 : Constant  Value=hex2dec('FFFF')  OutDataTypeStr=uint16
  Constant6 : Constant  Value=32  OutDataTypeStr=int32
  Constant7 : Constant  Value=10  OutDataTypeStr=int32
  Constant8 : Constant  Value=64  OutDataTypeStr=int32
  Constant9 : Constant  Value=100  OutDataTypeStr=uint32
  Display Touchscreen : Raptor_display_lib/Touchscreen/Display Touchscreen
      settings: SourceProductName=Raptor Display Library
  Logical Operator : Logic  Inputs=5  IconShape=distinctive  AllPortsSameDT=off  OutDataTypeStr=boolean
  Relational Operator : RelationalOperator  OutDataTypeStr=boolean  InputSameDT=off
  Relational Operator1 : RelationalOperator  OutDataTypeStr=boolean  InputSameDT=off
  Relational Operator2 : RelationalOperator  Operator=<=  OutDataTypeStr=boolean  InputSameDT=off
  Relational Operator3 : RelationalOperator  Operator=<=  OutDataTypeStr=boolean  InputSameDT=off
  Switch1 : Switch  Criteria=u2 ~= 0  SaturateOnIntegerOverflow=off  InputSameDT=off
  Switch2 : Switch  Criteria=u2 ~= 0  SaturateOnIntegerOverflow=off  InputSameDT=off
  Triggered Subsystem : Subsystem  TreatAsAtomicUnit=on
  Unit Delay : UnitDelay  SampleTime=-1  HasFrameUpgradeWarning=on
  Unit Delay1 : UnitDelay  InitialCondition=1  SampleTime=-1  HasFrameUpgradeWarning=on
  Unit Delay2 : UnitDelay  SampleTime=-1  HasFrameUpgradeWarning=on
  display_draw_image : Raptor_display_lib/Drawing Functions/display_draw_image  imagePort=off  imageFile=toggle_frame.png  opacityPort=off  opacity=100  drawMode=Draw Entire Image  alpha=Draw as Transparent  layer=Background  drawModeXY=Top Left  pnPort=on
      settings: SourceProductName=Raptor Display Library
  display_draw_text : Raptor_display_lib/Drawing Functions/display_draw_text  textPort=off  textVal='On'  colorPort=on  col=8410  opacity=100  font=Future  fontFile=''  heightPort=off  height=20  hAlign=Center  vAlign=Top  spacing=0  layer=Background  pnPort=off
      settings: SourceProductName=Raptor Display Library
  display_draw_text1 : Raptor_display_lib/Drawing Functions/display_draw_text  textPort=off  textVal='Off'  colorPort=on  col=FFFF  opacity=100  font=Future  fontFile=''  heightPort=off  height=20  hAlign=Center  vAlign=Top  spacing=0  layer=Background  pnPort=off
      settings: SourceProductName=Raptor Display Library
  next : Outport  VectorParamsAs1DForOutWhenUnconnected=off
  out : Outport  Port=2  VectorParamsAs1DForOutWhenUnconnected=off
  wires:
  x/1 -> Add/1, Relational Operator/2, Add2/1, display_draw_image/2
  Display Touchscreen/2 -> Relational Operator/1, Relational Operator2/1
  Display Touchscreen/3 -> Relational Operator1/1, Relational Operator3/1
  y/1 -> Add1/1, Relational Operator1/2, Add3/1, display_draw_image/3
  Constant/1 -> Add/2
  Constant1/1 -> Add1/2
  Add/1 -> Relational Operator2/2
  Add1/1 -> Relational Operator3/2
  Relational Operator3/1 -> Logical Operator/5
  Relational Operator1/1 -> Logical Operator/4
  Relational Operator2/1 -> Logical Operator/3
  Relational Operator/1 -> Logical Operator/2
  Display Touchscreen/1 -> Logical Operator/1
  Unit Delay1/1 -> Unit Delay2/1
  Unit Delay/1 -> Unit Delay1/1
  Logical Operator/1 -> Unit Delay/1
  Unit Delay2/1 -> Triggered Subsystem/Trigger
  prev/1 -> display_draw_image/1
  display_draw_image/1 -> next/1
  Triggered Subsystem/1(Out1) -> Switch1/2, Switch2/2, out/1
  Switch1/1 -> display_draw_text/3
  Switch2/1 -> display_draw_text1/3
  Constant2/1 -> Switch2/1
  Constant4/1 -> Switch1/3
  Constant3/1 -> Switch2/3
  Constant5/1 -> Switch1/1
  Constant6/1 -> Add2/2
  Add2/1 -> Add4/1, display_draw_text/1
  Constant7/1 -> Add3/2
  Add3/1 -> display_draw_text/2, display_draw_text1/2
  Constant8/1 -> Add4/2
  Add4/1 -> display_draw_text1/1
  Constant9/1 -> display_draw_text/4
  Constant10/1 -> display_draw_text1/4

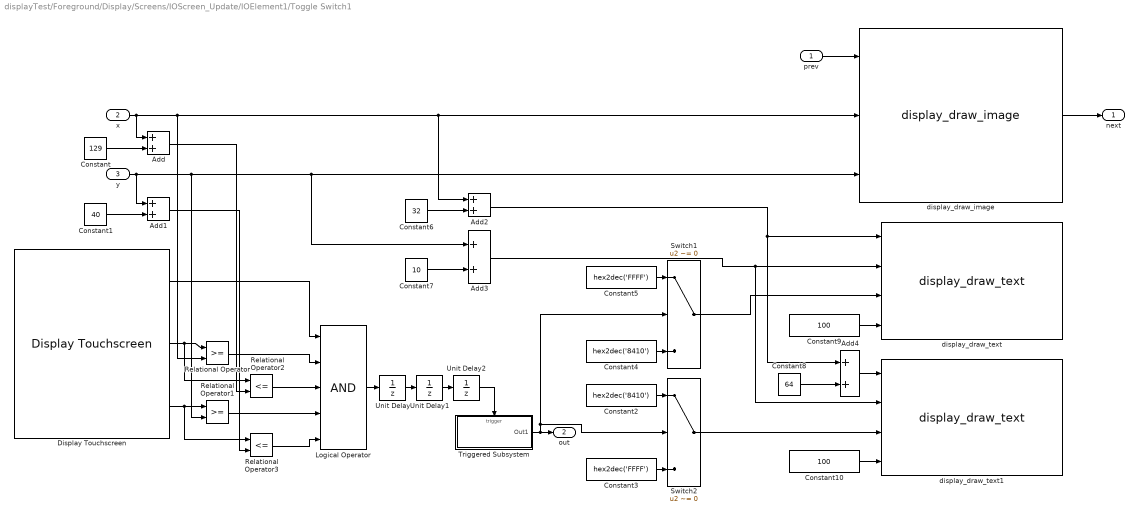
== system displayTest/Foreground/Display/Screens/IOScreen_Update/IOElement1/Toggle Switch1 ==
  prev : Inport
  x : Inport  Port=2
  y : Inport  Port=3
  Add{,1..4} (5 alike) : Sum
  Constant : Constant  Value=129
  Constant1 : Constant  Value=40
  Constant10 : Constant  Value=100  OutDataTypeStr=uint32
  Constant2 : Constant  Value=hex2dec('8410')  OutDataTypeStr=uint16
  Constant3 : Constant  Value=hex2dec('FFFF')  OutDataTypeStr=uint16
  Constant4 : Constant  Value=hex2dec('8410')  OutDataTypeStr=uint16
  Constant5 : Constant  Value=hex2dec('FFFF')  OutDataTypeStr=uint16
  Constant6 : Constant  Value=32  OutDataTypeStr=int32
  Constant7 : Constant  Value=10  OutDataTypeStr=int32
  Constant8 : Constant  Value=64  OutDataTypeStr=int32
  Constant9 : Constant  Value=100  OutDataTypeStr=uint32
  Display Touchscreen : Raptor_display_lib/Touchscreen/Display Touchscreen
      settings: SourceProductName=Raptor Display Library
  Logical Operator : Logic  Inputs=5  IconShape=distinctive  AllPortsSameDT=off  OutDataTypeStr=boolean
  Relational Operator : RelationalOperator  OutDataTypeStr=boolean  InputSameDT=off
  Relational Operator1 : RelationalOperator  OutDataTypeStr=boolean  InputSameDT=off
  Relational Operator2 : RelationalOperator  Operator=<=  OutDataTypeStr=boolean  InputSameDT=off
  Relational Operator3 : RelationalOperator  Operator=<=  OutDataTypeStr=boolean  InputSameDT=off
  Switch1 : Switch  Criteria=u2 ~= 0  SaturateOnIntegerOverflow=off  InputSameDT=off
  Switch2 : Switch  Criteria=u2 ~= 0  SaturateOnIntegerOverflow=off  InputSameDT=off
  Triggered Subsystem : Subsystem  TreatAsAtomicUnit=on
  Unit Delay : UnitDelay  SampleTime=-1  HasFrameUpgradeWarning=on
  Unit Delay1 : UnitDelay  InitialCondition=1  SampleTime=-1  HasFrameUpgradeWarning=on
  Unit Delay2 : UnitDelay  SampleTime=-1  HasFrameUpgradeWarning=on
  display_draw_image : Raptor_display_lib/Drawing Functions/display_draw_image  imagePort=off  imageFile=toggle_frame.png  opacityPort=off  opacity=100  drawMode=Draw Entire Image  alpha=Draw as Transparent  layer=Background  drawModeXY=Top Left  pnPort=on
      settings: SourceProductName=Raptor Display Library
  display_draw_text : Raptor_display_lib/Drawing Functions/display_draw_text  textPort=off  textVal='On'  colorPort=on  col=8410  opacity=100  font=Future  fontFile=''  heightPort=off  height=20  hAlign=Center  vAlign=Top  spacing=0  layer=Background  pnPort=off
      settings: SourceProductName=Raptor Display Library
  display_draw_text1 : Raptor_display_lib/Drawing Functions/display_draw_text  textPort=off  textVal='Off'  colorPort=on  col=FFFF  opacity=100  font=Future  fontFile=''  heightPort=off  height=20  hAlign=Center  vAlign=Top  spacing=0  layer=Background  pnPort=off
      settings: SourceProductName=Raptor Display Library
  next : Outport  VectorParamsAs1DForOutWhenUnconnected=off
  out : Outport  Port=2  VectorParamsAs1DForOutWhenUnconnected=off
  wires:
  x/1 -> Add/1, Relational Operator/2, Add2/1, display_draw_image/2
  Display Touchscreen/2 -> Relational Operator/1, Relational Operator2/1
  Display Touchscreen/3 -> Relational Operator1/1, Relational Operator3/1
  y/1 -> Add1/1, Relational Operator1/2, Add3/1, display_draw_image/3
  Constant/1 -> Add/2
  Constant1/1 -> Add1/2
  Add/1 -> Relational Operator2/2
  Add1/1 -> Relational Operator3/2
  Relational Operator3/1 -> Logical Operator/5
  Relational Operator1/1 -> Logical Operator/4
  Relational Operator2/1 -> Logical Operator/3
  Relational Operator/1 -> Logical Operator/2
  Display Touchscreen/1 -> Logical Operator/1
  Unit Delay1/1 -> Unit Delay2/1
  Unit Delay/1 -> Unit Delay1/1
  Logical Operator/1 -> Unit Delay/1
  Unit Delay2/1 -> Triggered Subsystem/Trigger
  prev/1 -> display_draw_image/1
  display_draw_image/1 -> next/1
  Triggered Subsystem/1(Out1) -> Switch1/2, Switch2/2, out/1
  Switch1/1 -> display_draw_text/3
  Switch2/1 -> display_draw_text1/3
  Constant2/1 -> Switch2/1
  Constant4/1 -> Switch1/3
  Constant3/1 -> Switch2/3
  Constant5/1 -> Switch1/1
  Constant6/1 -> Add2/2
  Add2/1 -> Add4/1, display_draw_text/1
  Constant7/1 -> Add3/2
  Add3/1 -> display_draw_text/2, display_draw_text1/2
  Constant8/1 -> Add4/2
  Add4/1 -> display_draw_text1/1
  Constant9/1 -> display_draw_text/4
  Constant10/1 -> display_draw_text1/4

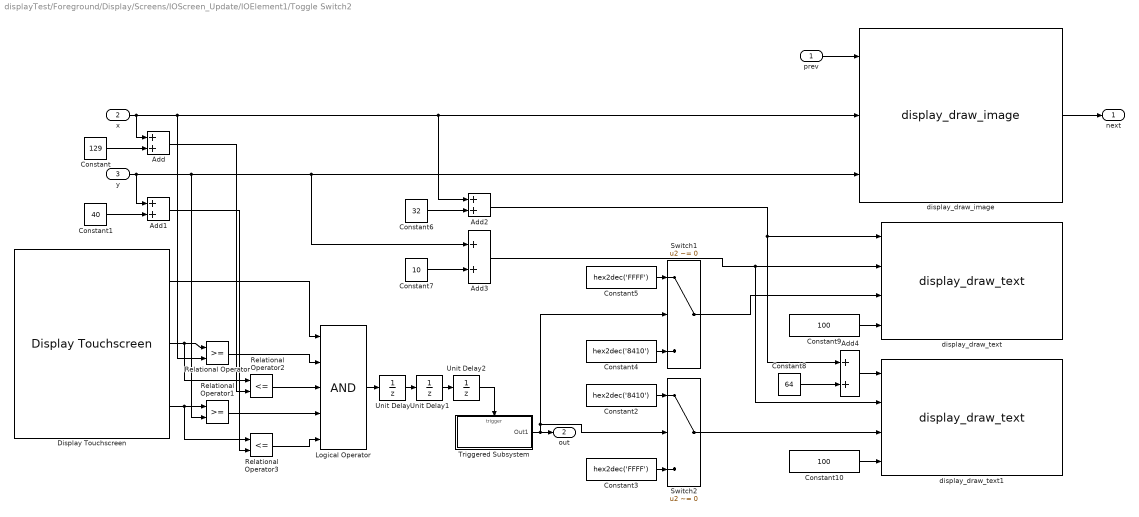
== system displayTest/Foreground/Display/Screens/IOScreen_Update/IOElement1/Toggle Switch2 ==
  prev : Inport
  x : Inport  Port=2
  y : Inport  Port=3
  Add{,1..4} (5 alike) : Sum
  Constant : Constant  Value=129
  Constant1 : Constant  Value=40
  Constant10 : Constant  Value=100  OutDataTypeStr=uint32
  Constant2 : Constant  Value=hex2dec('8410')  OutDataTypeStr=uint16
  Constant3 : Constant  Value=hex2dec('FFFF')  OutDataTypeStr=uint16
  Constant4 : Constant  Value=hex2dec('8410')  OutDataTypeStr=uint16
  Constant5 : Constant  Value=hex2dec('FFFF')  OutDataTypeStr=uint16
  Constant6 : Constant  Value=32  OutDataTypeStr=int32
  Constant7 : Constant  Value=10  OutDataTypeStr=int32
  Constant8 : Constant  Value=64  OutDataTypeStr=int32
  Constant9 : Constant  Value=100  OutDataTypeStr=uint32
  Display Touchscreen : Raptor_display_lib/Touchscreen/Display Touchscreen
      settings: SourceProductName=Raptor Display Library
  Logical Operator : Logic  Inputs=5  IconShape=distinctive  AllPortsSameDT=off  OutDataTypeStr=boolean
  Relational Operator : RelationalOperator  OutDataTypeStr=boolean  InputSameDT=off
  Relational Operator1 : RelationalOperator  OutDataTypeStr=boolean  InputSameDT=off
  Relational Operator2 : RelationalOperator  Operator=<=  OutDataTypeStr=boolean  InputSameDT=off
  Relational Operator3 : RelationalOperator  Operator=<=  OutDataTypeStr=boolean  InputSameDT=off
  Switch1 : Switch  Criteria=u2 ~= 0  SaturateOnIntegerOverflow=off  InputSameDT=off
  Switch2 : Switch  Criteria=u2 ~= 0  SaturateOnIntegerOverflow=off  InputSameDT=off
  Triggered Subsystem : Subsystem  TreatAsAtomicUnit=on
  Unit Delay : UnitDelay  SampleTime=-1  HasFrameUpgradeWarning=on
  Unit Delay1 : UnitDelay  InitialCondition=1  SampleTime=-1  HasFrameUpgradeWarning=on
  Unit Delay2 : UnitDelay  SampleTime=-1  HasFrameUpgradeWarning=on
  display_draw_image : Raptor_display_lib/Drawing Functions/display_draw_image  imagePort=off  imageFile=toggle_frame.png  opacityPort=off  opacity=100  drawMode=Draw Entire Image  alpha=Draw as Transparent  layer=Background  drawModeXY=Top Left  pnPort=on
      settings: SourceProductName=Raptor Display Library
  display_draw_text : Raptor_display_lib/Drawing Functions/display_draw_text  textPort=off  textVal='On'  colorPort=on  col=8410  opacity=100  font=Future  fontFile=''  heightPort=off  height=20  hAlign=Center  vAlign=Top  spacing=0  layer=Background  pnPort=off
      settings: SourceProductName=Raptor Display Library
  display_draw_text1 : Raptor_display_lib/Drawing Functions/display_draw_text  textPort=off  textVal='Off'  colorPort=on  col=FFFF  opacity=100  font=Future  fontFile=''  heightPort=off  height=20  hAlign=Center  vAlign=Top  spacing=0  layer=Background  pnPort=off
      settings: SourceProductName=Raptor Display Library
  next : Outport  VectorParamsAs1DForOutWhenUnconnected=off
  out : Outport  Port=2  VectorParamsAs1DForOutWhenUnconnected=off
  wires:
  Constant10/1 -> display_draw_text1/4
  Constant9/1 -> display_draw_text/4
  Add4/1 -> display_draw_text1/1
  Constant8/1 -> Add4/2
  Add3/1 -> display_draw_text1/2, display_draw_text/2
  Constant7/1 -> Add3/2
  Add2/1 -> display_draw_text/1, Add4/1
  Constant6/1 -> Add2/2
  Constant5/1 -> Switch1/1
  Constant3/1 -> Switch2/3
  Constant4/1 -> Switch1/3
  Constant2/1 -> Switch2/1
  Switch2/1 -> display_draw_text1/3
  Switch1/1 -> display_draw_text/3
  Triggered Subsystem/1(Out1) -> out/1, Switch2/2, Switch1/2
  display_draw_image/1 -> next/1
  prev/1 -> display_draw_image/1
  Unit Delay2/1 -> Triggered Subsystem/Trigger
  Logical Operator/1 -> Unit Delay/1
  Unit Delay/1 -> Unit Delay1/1
  Unit Delay1/1 -> Unit Delay2/1
  Display Touchscreen/1 -> Logical Operator/1
  Relational Operator/1 -> Logical Operator/2
  Relational Operator2/1 -> Logical Operator/3
  Relational Operator1/1 -> Logical Operator/4
  Relational Operator3/1 -> Logical Operator/5
  Add1/1 -> Relational Operator3/2
  Add/1 -> Relational Operator2/2
  Constant1/1 -> Add1/2
  Constant/1 -> Add/2
  y/1 -> display_draw_image/3, Add3/1, Relational Operator1/2, Add1/1
  Display Touchscreen/3 -> Relational Operator3/1, Relational Operator1/1
  Display Touchscreen/2 -> Relational Operator2/1, Relational Operator/1
  x/1 -> display_draw_image/2, Add2/1, Relational Operator/2, Add/1

== system displayTest/Foreground/Display/Screens/Navigation/Go Left/About ==
  Action Port : ActionPort  ActionPortLabel=case [ 4 ]:
  display_goto_screen : Raptor_display_lib/Screen Functions/display_goto_screen  screenPort=off  ScreenName='MainScreen'
      settings: SourceProductName=Raptor Display Library

== system displayTest/Foreground/Display/Screens/Navigation/Go Left/DataLog ==
  Action Port : ActionPort  ActionPortLabel=case [ 3 ]:
  display_goto_screen : Raptor_display_lib/Screen Functions/display_goto_screen  screenPort=off  ScreenName='AboutScreen'
      settings: SourceProductName=Raptor Display Library

== system displayTest/Foreground/Display/Screens/Navigation/Go Left/Default ==
  Action Port : ActionPort  ActionPortLabel=default:
  display_goto_screen : Raptor_display_lib/Screen Functions/display_goto_screen  screenPort=off  ScreenName='MainScreen'
      settings: SourceProductName=Raptor Display Library

== system displayTest/Foreground/Display/Screens/Navigation/Go Left/IO ==
  Action Port : ActionPort  ActionPortLabel=case [ 2 ]:
  display_goto_screen : Raptor_display_lib/Screen Functions/display_goto_screen  screenPort=off  ScreenName='DataLogScreen'
      settings: SourceProductName=Raptor Display Library

== system displayTest/Foreground/Display/Screens/Navigation/Go Left/Main ==
  Action Port : ActionPort  ActionPortLabel=case [ 1 ]:
  display_goto_screen : Raptor_display_lib/Screen Functions/display_goto_screen  screenPort=off  ScreenName='IOScreen'
      settings: SourceProductName=Raptor Display Library

== system displayTest/Foreground/Display/Screens/Navigation/Go Right/About ==
  Action Port : ActionPort  ActionPortLabel=case [ 4 ]:
  display_goto_screen : Raptor_display_lib/Screen Functions/display_goto_screen  screenPort=off  ScreenName='DataLogScreen'
      settings: SourceProductName=Raptor Display Library

== system displayTest/Foreground/Display/Screens/Navigation/Go Right/DataLog ==
  Action Port : ActionPort  ActionPortLabel=case [ 3 ]:
  display_goto_screen : Raptor_display_lib/Screen Functions/display_goto_screen  screenPort=off  ScreenName='IOScreen'
      settings: SourceProductName=Raptor Display Library

== system displayTest/Foreground/Display/Screens/Navigation/Go Right/Default ==
  Action Port : ActionPort  ActionPortLabel=default:
  display_goto_screen : Raptor_display_lib/Screen Functions/display_goto_screen  screenPort=off  ScreenName='MainScreen'
      settings: SourceProductName=Raptor Display Library
